simulink model "Load_Freq_Ctrl"  (R2014b)
settings: Solver=ode45  StartTime=0.0  StopTime=10.0  RelTol=1e-3
libraries: powerlib x1
settings Model: Creator=Student  LastModifiedBy=Bismillah!

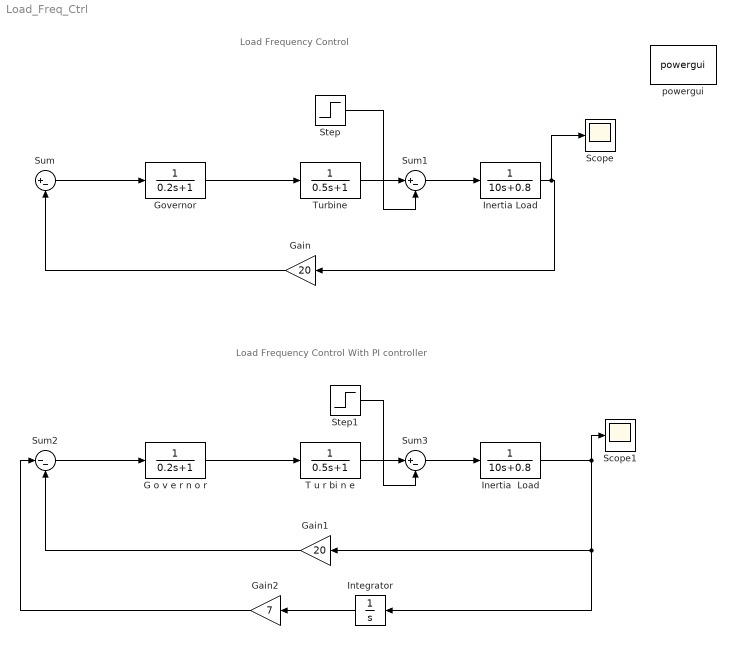
== system Load_Freq_Ctrl ==
  note: Load Frequency Control With PI controller
  note: Load Frequency Control
  G o v e r n o r : TransferFcn  Denominator=[0.2 1]
  Gain : Gain  Gain=20
  Gain1 : Gain  Gain=20
  Gain2 : Gain  Gain=7
  Governor : TransferFcn  Denominator=[0.2 1]
  Inertia  Load : TransferFcn  Denominator=[10 0.8]
  Inertia Load : TransferFcn  Denominator=[10 0.8]
  Integrator : Integrator
  Scope : Scope
  Scope1 : Scope
  Step : Step  Time=0  After=0.2  SampleTime=0
  Step1 : Step  Time=0  After=0.2  SampleTime=0
  Sum : Sum  Inputs=|+-
  Sum1 : Sum  Inputs=|+-
  Sum2 : Sum  Inputs=|--
  Sum3 : Sum  Inputs=|+-
  T u r bi n e : TransferFcn  Denominator=[0.5 1]
  Turbine : TransferFcn  Denominator=[0.5 1]
  powergui : powerlib/powergui  Priority=1  SimulationMode=Continuous  SolverType=Tustin/Backward Euler (TBE)  SampleTime=50e-6  frequency=60  SPID=off  DisableSnubberDevices=off  DisableRonSwitches=off  DisableVfSwitches=off  SwTol=0  DisplayEquations=off  Interpol=off  methode=off  Ts=100  frequencyindice=60  Pbase=100e6  ErrMax=1e-4  Iterations=50  UnitsV=kV  UnitsW=MW  FunctionMessages=off  echomessages=off  HookPort=off  EnableUseOfTLC=off  x0status=blocks  RestoreLinks=warning  ResistiveCurrentMeasurement=off  Frange=[0:2:500]  Ylog=off  Xlog=on  ShowGrid=off  save=off  variable=ZData  structure=0  ZoomFFT=off  StartTime=0.0  cycles=1  DisplayStyle=1  fundamental=60  FreqAxis=off  MaxFrequency=1000  frequencyindicesteady=1  RmsSteady=1  display=off
  wires:
  Sum/1 -> Governor/1
  Governor/1 -> Turbine/1
  Turbine/1 -> Sum1/1
  Step/1 -> Sum1/2
  Sum1/1 -> Inertia Load/1
  Inertia Load/1 -> Scope/1, Gain/1
  Gain/1 -> Sum/2
  Sum2/1 -> G o v e r n o r/1
  G o v e r n o r/1 -> T u r bi n e/1
  T u r bi n e/1 -> Sum3/1
  Step1/1 -> Sum3/2
  Sum3/1 -> Inertia  Load/1
  Inertia  Load/1 -> Integrator/1, Gain1/1, Scope1/1
  Gain1/1 -> Sum2/2
  Gain2/1 -> Sum2/1
  Integrator/1 -> Gain2/1
